simulink model "multilevel_inverter"  (R2020a)
settings: Solver=VariableStepAuto  StartTime=0.0  StopTime=0.1  RelTol=1e-3
libraries: powerlib x12, simulink x4
settings Model: Creator=Reaga  LastModifiedBy=Reaga
settings DebuggingCC: UnconnectedInputMsg=none  UnconnectedOutputMsg=none  UnconnectedLineMsg=none
settings ModelReferenceCC: EnableRefExpFcnMdlSchedulingChecks=off
settings RTWCC: Description=Generic Real-Time Target
settings ConfigComp: CovBoundaryAbsTol=1.0e-5

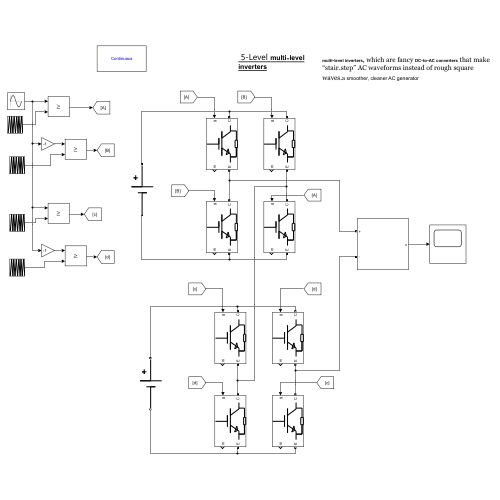
[thumbnail: Simulink's stored preview of the top-level diagram]
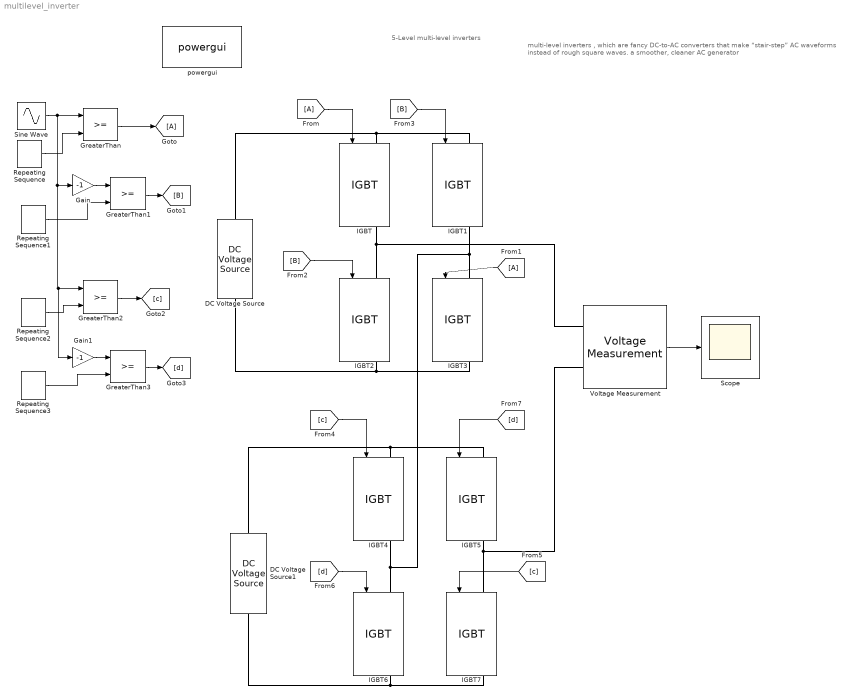
== system multilevel_inverter ==
  note: 5-Level multi‑level inverters
  note: multi‑level inverters , which are fancy DC‑to‑AC converters that make “stair‑step” AC waveforms instead of rough square waves. a smoother, cleaner AC generator
  DC Voltage Source : powerlib/Electrical Sources/DC Voltage Source  Amplitude=100  Measurements=None
  DC Voltage Source1 : powerlib/Electrical Sources/DC Voltage Source  Amplitude=100  Measurements=None
  Gain : Gain  Gain=-1
  Gain1 : Gain  Gain=-1
  GreaterThan{,1..3} (4 alike) : RelationalOperator  OutDataTypeStr=boolean  RndMeth=Simplest
  IGBT{,1..7} (8 alike) : powerlib/Power Electronics/IGBT  Ron=0.001  Lon=0  Vf=1  Tf=1e-6  Tt=2e-6  IC=0  Rs=1e5  Cs=inf  Measurements=on
  Repeating Sequence : simulink/Sources/Repeating Sequence  rep_seq_t=[0 1e-3 0.002 0.003 0.004]  rep_seq_y=[0 1 0 1 0]
  Repeating Sequence1 : simulink/Sources/Repeating Sequence  rep_seq_t=[0 1e-3 0.002 0.003 0.004]  rep_seq_y=[0 1 0 1 0]
  Repeating Sequence2 : simulink/Sources/Repeating Sequence  rep_seq_t=[0 1e-3 0.002 0.003 0.004]  rep_seq_y=[1 2 1 2 1]
  Repeating Sequence3 : simulink/Sources/Repeating Sequence  rep_seq_t=[0 1e-3 0.002 0.003 0.004]  rep_seq_y=[1 2 1 2 1]
  Scope : Scope
  Sine Wave : Sin  Amplitude=2  Frequency=2*50*pi  SampleTime=0
  Voltage Measurement : powerlib/Measurements/Voltage Measurement  PhasorSimulation=off  OutputType=Complex  PSBequivalent=0
  powergui : powerlib/powergui  Priority=1  SimulationMode=Continuous  SampleTime=50e-6  frequency=60  Iterations=50  frequencyindice=0  Pbase=100e6  ErrMax=1e-4  UnitsV=kV  UnitsW=MW  buscounter=0  FunctionMessages=off  echomessages=off  EnableUseOfTLC=off  CurrentSourceSwitches=off  DisableSnubberDevices=off  DisableRonSwitches=off  DisableVfSwitches=off  DisplayEquations=off  AutomaticDiscreteSolvers=off  SolverType=Tustin/Backward Euler (TBE)  Interpol=off  ExternalGateDelay=off  methode=off  Ts=100  x0status=blocks  SPID=on  SwTol=0  HookPort=off  NonlinearTolerance=1e-4  nMaxIteration=100  ContinueOnMaxIteration=off  RestoreLinks=warning  ResistiveCurrentMeasurement=off  Frange=[0:2:500]  Ylog=off  Xlog=on  ShowGrid=off  save=off  variable=ZData  structure=0  ZoomFFT=off  StartTime=0.0  cycles=1  DisplayStyle=1  fundamental=60  FreqAxis=off  MaxFrequency=1000  frequencyindicesteady=1  RmsSteady=1  display=off
  wires:
  [A] -> IGBT/1
  [A] -> IGBT3/1
  [B] -> IGBT2/1
  [B] -> IGBT1/1
  [c] -> IGBT4/1
  [c] -> IGBT7/1
  [d] -> IGBT6/1
  [d] -> IGBT5/1
  Voltage Measurement/1 -> Scope/1
  Sine Wave/1 -> Gain1/1, GreaterThan2/1, Gain/1, GreaterThan/1
  Repeating Sequence/1 -> GreaterThan/2
  GreaterThan/1 -> [A]
  Gain/1 -> GreaterThan1/1
  Repeating Sequence1/1 -> GreaterThan1/2
  GreaterThan1/1 -> [B]
  Repeating Sequence2/1 -> GreaterThan2/2
  GreaterThan2/1 -> [c]
  Gain1/1 -> GreaterThan3/1
  Repeating Sequence3/1 -> GreaterThan3/2
  GreaterThan3/1 -> [d]
  connections:
  IGBT/RConn1 -- Voltage Measurement/LConn1 -- IGBT2/LConn1
  DC Voltage Source/RConn1 -- IGBT1/LConn1 -- IGBT/LConn1
  DC Voltage Source/LConn1 -- IGBT3/RConn1 -- IGBT2/RConn1
  IGBT6/RConn1 -- DC Voltage Source1/LConn1 -- IGBT7/RConn1
  DC Voltage Source1/RConn1 -- IGBT5/LConn1 -- IGBT4/LConn1
  IGBT3/LConn1 -- IGBT6/LConn1 -- IGBT4/RConn1 -- IGBT1/RConn1
  IGBT7/LConn1 -- Voltage Measurement/LConn2 -- IGBT5/RConn1
